simulink model "part2_datalog1_oldsimulink"  (R2018a)
settings: Solver=FixedStepAuto  StartTime=0.0  StopTime=count  FixedStep=1  RelTol=1e-3
libraries: simulink x2
settings Model: Creator=pdranishnikov5258  LastModifiedBy=pete404

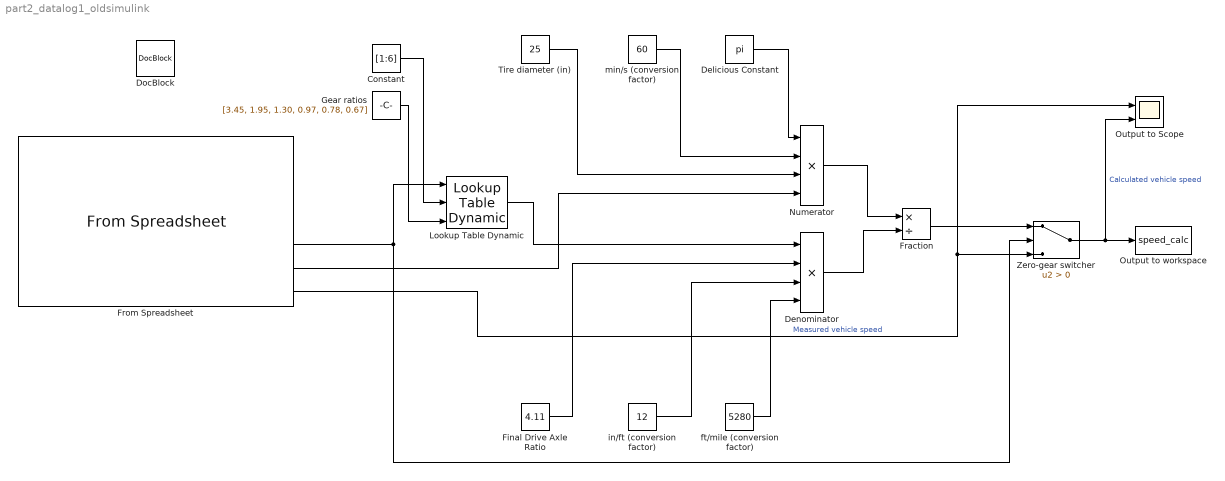
== system part2_datalog1_oldsimulink ==
  Constant : Constant  Value=[1:6]
  Delicious Constant : Constant  Value=pi
  Denominator : Product  Inputs=4
  DocBlock : simulink/Model-Wide Utilities/DocBlock  DocumentType=Text
      content=|
      | Type your documentation here:
      |
      | Author: Peter A. Dranishnikov
      | Lab #: 5
      | Course: EEL 4685C
      | Due date: March 19th, Spring 2019
  Final Drive Axle Ratio : Constant  Value=4.11
  Fraction : Product  Inputs=*/
  From Spreadsheet : FromSpreadsheet  FileName=datalog1.xlsx  SheetName=datalog1
  Gear ratios : Constant  Value=[3.45, 1.95, 1.30, 0.97, 0.78, 0.67]
  Lookup Table Dynamic : simulink/Lookup Tables/Lookup Table Dynamic  LookUpMeth=Interpolation-Use End Values  OutDataType=fixdt('double')  OutScaling=[]  OutputDataTypeScalingMode=Specify via dialog  OutDataTypeStr=double  DoSatur=off
      settings: SourceProductName=Simulink
  Numerator : Product  Inputs=4
  Output to Scope : Scope  NumInputPorts=2
  Output to workspace : ToWorkspace  VariableName=speed_calc  SampleTime=-1
      settings: Save2DSignal=2-D array (concatenate along first dimension)
  Tire diameter (in) : Constant  Value=25
  Zero-gear switcher : Switch  Criteria=u2 > Threshold
  ft/mile (conversion factor) : Constant  Value=5280
  in/ft (conversion factor) : Constant  Value=12
  min/s (conversion factor) : Constant  Value=60
  wires:
  Delicious Constant/1 -> Numerator/1
  Numerator/1 -> Fraction/1
  Denominator/1 -> Fraction/2
  ft/mile (conversion factor)/1 -> Denominator/4
  in/ft (conversion factor)/1 -> Denominator/3
  min/s (conversion factor)/1 -> Numerator/2
  From Spreadsheet/6 -> Numerator/4
  Tire diameter (in)/1 -> Numerator/3
  Lookup Table Dynamic/1 -> Denominator/1
  From Spreadsheet/5 -> Zero-gear switcher/2, Lookup Table Dynamic/1
  Constant/1 -> Lookup Table Dynamic/2
  Gear ratios/1 -> Lookup Table Dynamic/3
  From Spreadsheet/7 -> Output to Scope/1, Zero-gear switcher/3  "Measured vehicle speed"
  Fraction/1 -> Zero-gear switcher/1
  Final Drive Axle Ratio/1 -> Denominator/2
  Zero-gear switcher/1 -> Output to Scope/2, Output to workspace/1  "Calculated vehicle speed"
